simulink model "HAITEC"  (R2013a)
settings: Solver=FixedStepDiscrete  StartTime=0.0  StopTime=240.0  FixedStep=0.1  RelTol=1e-3
InitFcn:
  | close all;
  | s=dbstatus;
  | save('myBreakpoints.mat', 's');
  | clear all;
  | load('myBreakpoints.mat');
  | VelocityListBus();
  | YawRateListBus();
  | ObstacleListBus();
  | ObjectListBus();
  | TrackListBus();
  | dbstop(s);
  | 
  | 
  | %===========================
  | % PROVIDE PATH TO BST STREAM
  | %===========================
  | %filepath = 'HAITECObjects.bst';
  | %filepath = 'HAITECTargets.bst';
  | %filepath = 'ObjectsData.bst';
  | filepath = 'Stream 20160506 16_33_31_434.bst';
  | %===========================
  | % DO NOT CHANGE THE LINES BELOW
  | %===========================
  | 
  | uintfilepath = uint8(filepath);
settings Model: Creator=Admin  LastModifiedBy=kawa
settings DebuggingCC: FrameProcessingCompatibilityMsg=error  StateNameClashWarn=none
settings SFSimCC: SimParseCustomCode=off
settings GRTTargetCC: CodeReplacementLibrary=C89/C90 (ANSI)

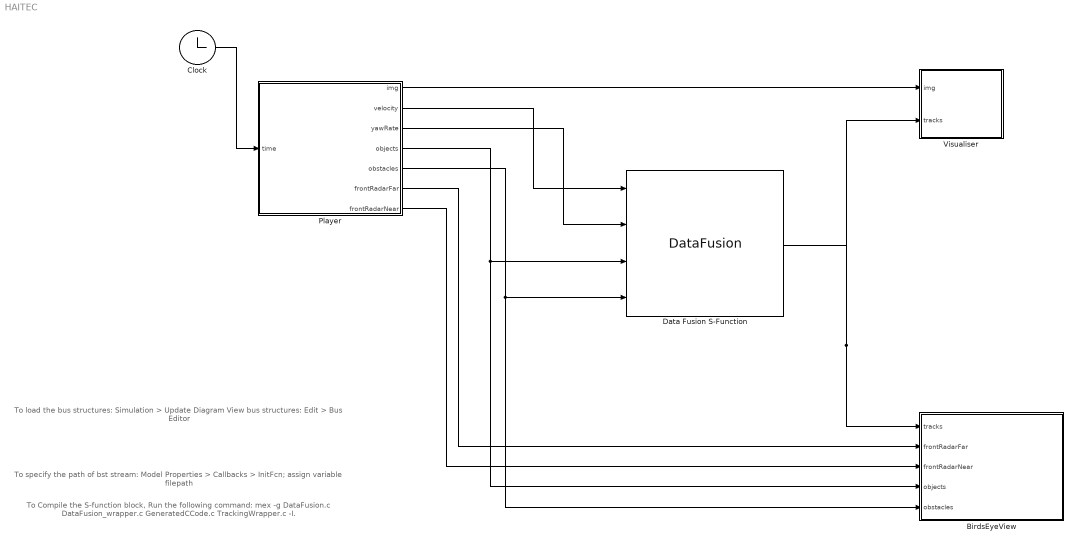
== system HAITEC ==
  note: To load the bus structures:
      | Simulation > Update Diagram
      |
      | View bus structures:
      | Edit > Bus Editor
  note: To specify the path of bst stream:
      | Model Properties > Callbacks > InitFcn; assign variable filepath
  note: To Compile the S-function block, Run the following command:
      | mex -g DataFusion.c DataFusion_wrapper.c GeneratedCCode.c TrackingWrapper.c -I.
  BirdsEyeView : MATLAB Function  TreatAsAtomicUnit=on
  Clock : Clock
  Data Fusion S-Function : S-Function  InitFcn=try, set_param(gcb,'FunctionName','DataFusion'), end  FunctionName=DataFusion  SFunctionModules=DataFusion_wrapper TrackingWrapper GeneratedCCode  EnableBusSupport=off  mask(S-Function Builder){}
      mask help: Simulink:masks:SFunctionBuilder_MD
      mask init:
      | val = [[.9  0.75 0.75 1 1 .9 .9 1]',[1 1 0.75 0.75 .9 .9 1 .9]'];try , sys = get_param(gcb,'SfunBuilderFcnName');if isempty(sys), sys = get_param(gcb,'FunctionName'); end,catch, sys = get_param(gcb,'FunctionName'); end
      settings: CopyFcn=set_param(gcbh,'LinkStatus','none')  PreSaveFcn=try, set_param(gcb,'FunctionName','DataFusion'), end  OpenFcn=sfunctionwizard(gcbh)
      mask Display: plot(val(:,1),val(:,2)),disp(sys), port_label('input',1,'velocity'), port_label('input',2,'yawRate'), port_label('input',3,'objects'), port_label('input',4,'obstacles'), port_label('output',1,'tracks')
  Player : MATLAB Function  TreatAsAtomicUnit=on
  Visualiser : MATLAB Function  TreatAsAtomicUnit=on
  wires:
  Clock/1 -> Player/1(time)
  Player/6(frontRadarFar) -> BirdsEyeView/2(frontRadarFar)
  Player/7(frontRadarNear) -> BirdsEyeView/3(frontRadarNear)
  Player/1(img) -> Visualiser/1(img)
  Player/4(objects) -> Data Fusion S-Function/3, BirdsEyeView/4(objects)
  Player/5(obstacles) -> BirdsEyeView/5(obstacles), Data Fusion S-Function/4
  Player/2(velocity) -> Data Fusion S-Function/1
  Player/3(yawRate) -> Data Fusion S-Function/2
  Data Fusion S-Function/1 -> BirdsEyeView/1(tracks), Visualiser/2(tracks)

== matlab function HAITEC/Visualiser ==
  data: img input; tracks input Bus: TrackList size=1
function Visualiser(img, tracks)
coder.extrinsic('plotImage','plotTracksInImage','imshow');
coder.extrinsic('delete');
coder.extrinsic('image');

persistent imageHandle;
persistent figureHandle;

if isempty(imageHandle)       
    figureHandle = subplot(1,2,2);
    imageHandle = image(img,'Parent', figureHandle);
    set(gca,'visible','off');
    hold on;
end
plotImage(img, imageHandle);
plotTracksInImage(tracks, figureHandle);

end

== matlab function HAITEC/Player ==
  data: time input; img output; velocity output Bus: VelocityList size=1; uintfilepath parameter; yawRate output Bus: YawRateList size=1; objects output Bus: ObjectList size=1; obstacles output Bus: ObstacleList size=1; frontRadarFar output; frontRadarNear output
function [img, velocity, yawRate, objects, obstacles , frontRadarFar, frontRadarNear] = Player(time, uintfilepath)
coder.extrinsic('playData')
img = uint8(zeros(1200,1600,3));
frontRadarFar = NaN(90,4);
frontRadarNear = NaN(90,4);

velocity = struct('count', uint8(0), 'timestamp', uint32(zeros(30,1)), 'velocity', zeros(30,1)); 
yawRate = struct('count', uint8(0), 'timestamp', uint32(zeros(30,1)), 'yawRate', zeros(30,1));
objects = struct('timestampCount', uint8(0), 'timestamp', uint32(zeros(60,1)),...
    'objectCount', uint8(zeros(60,1)),'x', zeros(60,40), 'y', zeros(60,40),...
    'vx', zeros(60,40), 'vy', zeros(60,40), 'rollingCounter', uint8(zeros(60,40)),...
    'id', uint8(zeros(60,40)), 'ax', zeros(60,40), 'existenceProbability', zeros(60,40),...
    'dynamicProperty', uint8(zeros(60,40)), 'length', zeros(60,40), 'width', zeros(60,40),...
    'measurementStatus', uint8(zeros(60,40)) , 'rcsValue', zeros(60,40),...
    'obstacleProbability', zeros(60,40));
obstacles = struct('timestampCount', uint8(0), 'timestamp', uint32(zeros(60,1)),...
    'obstacleCount', uint8(zeros(60,1)), 'x', zeros(60,10), 'y', zeros(60,10),...
    'vx', zeros(60,10), 'vy', zeros(60,10), 'id', uint8(zeros(60,10)),...
    'obstacleType', uint8(zeros(60,10)),'obstacleStatus', uint8(zeros(60,10)),...
    'length', zeros(60,10), 'width', zeros(60,10),'angleRate', zeros(60,10),...
    'ax', zeros(60,10), 'angle', zeros(60,10), 'obstacleTimestamp', uint8(zeros(60,10)),...
    'cipvFlag', false(60,10));

[img, velocity, yawRate, frontRadarFar, frontRadarNear, objects, obstacles] = playData(time, uintfilepath);
end

== matlab function HAITEC/BirdsEyeView ==
  data: tracks input Bus: TrackList size=1; frontRadarFar input; frontRadarNear input; objects input Bus: ObjectList size=1; obstacles input Bus: ObstacleList size=1
function BirdsEyeView(tracks, frontRadarFar, frontRadarNear, objects, obstacles)
coder.extrinsic('plotData','plotSensorFOV');
persistent fig

if isempty(fig)       
    fig = subplot(1,2,1);
    set(gcf,'units','normalized','outerposition',[0 0 1 1]) %fullscreen
    axis equal
    axis([-10, 220, -40, 40]);
    title('Multiple Object Tracking')
    xlabel('x');
    ylabel('y');
    grid on;
    hold on;
    view([-90 90]) %rotate
    plotSensorFOV();
end

plotData(tracks, frontRadarFar, frontRadarNear, objects, obstacles, fig);

end
